simulink model "BatteryModel"  (R2018a)
settings: Solver=VariableStepAuto  StartTime=0.0  StopTime=10.0  RelTol=1e-3
values from neighbouring files (symbols this model uses):
  CN = 2.3    [Prj_5_BatteryModel.m]
  I = 2.3    [Prj_5_BatteryModel.m]
  OCV = data(:,2)    [Prj_5_BatteryModel.m]
  R_discharge = data(:,4)    [Prj_5_BatteryModel.m]
  SOC = data(:,1)    [Prj_5_BatteryModel.m]
settings Model: Creator=Admin  LastModifiedBy=Dpt_Mas

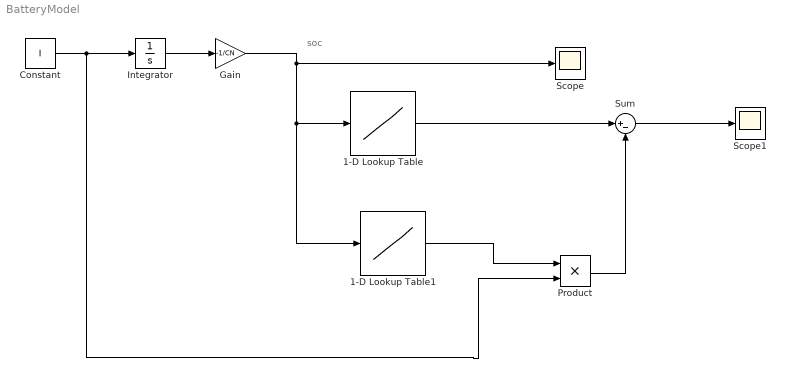
== system BatteryModel ==
  note: soc
  1-D Lookup Table : Lookup_n-D  NumberOfTableDimensions=1  BreakpointsForDimension1=SOC  Table=OCV  InternalRulePriority=Speed  RndMeth=Simplest  InputSameDT=on
  1-D Lookup Table1 : Lookup_n-D  NumberOfTableDimensions=1  BreakpointsForDimension1=SOC  Table=R_discharge  InternalRulePriority=Speed  RndMeth=Simplest  InputSameDT=on
  Constant : Constant  Value=I
  Gain : Gain  Gain=-1/CN
  Integrator : Integrator
  Product : Product
  Scope : Scope
  Scope1 : Scope
  Sum : Sum  Inputs=|+-
  wires:
  Constant/1 -> Product/2, Integrator/1
  Integrator/1 -> Gain/1
  Gain/1 -> Scope/1, 1-D Lookup Table1/1, 1-D Lookup Table/1
  Product/1 -> Sum/2
  1-D Lookup Table/1 -> Sum/1
  Sum/1 -> Scope1/1
  1-D Lookup Table1/1 -> Product/1
